simulink model "wb_poco_al_intfract_v00"  (Simulink 6.2)
settings: Solver=ode45  StartTime=0.0  StopTime=2^23  RelTol=1e-3
libraries: xbsIndex_r3 x705, xps_library x24, delay_lib x6, fft_library x2, pfb_library x1
(part 3 of 6)

== system wb_poco_al_intfract_v00/delay_wideband_prog0/delay_dp3 ==
  din : Inport  Port=1  LatchInput=off
  delay : Inport  Port=2  LatchInput=off
  AddSub : xbsIndex_r3/AddSub  mode=Subtraction  precision=User Defined  arith_type=Unsigned  n_bits=11  bin_pt=0  quantization=Truncate  overflow=Wrap  latency=1  explicit_period=off  period=1  use_carryin=off  use_carryout=off  en=off  dbl_ovrd=off  show_param=off  use_core=on  pipeline=off  use_rpm=on  gen_core=off
      settings: xl_area=[0, 0, 0, 0, 0, 0, 0]
  Constant2 : xbsIndex_r3/Constant  const=1  equ=P=C  arith_type=Boolean  n_bits=1  bin_pt=0  opselect=C  inp2=PCIN>>17  opr=+  inp1=P  carry=CIN  iostate=0  explicit_period=on  period=1  dbl_ovrd=off
  Constant4 : xbsIndex_r3/Constant  const=0  equ=P=C  arith_type=Boolean  n_bits=1  bin_pt=0  opselect=C  inp2=PCIN>>17  opr=+  inp1=P  carry=CIN  iostate=0  explicit_period=on  period=1  dbl_ovrd=off
  Dual Port RAM : S-Function  AncestorBlock=xbsIndex_r3/Dual Port RAM  FunctionName=xldpram  Parameters=sfcn_mwsv__  mask(Xilinx Dual Port Random Access Memory){depth=2048, initVector=0, write_mode_A=Read After Write, write_mode_B=Read After Write, latency=4, mem_collision=off, init_zero=on, explicit_period=off, period=1, dbl_ovrd=off, rst_a=off, init_a=0, rst_b=off, init_b=0, show_param=off, distributed_mem=off, use_rpm=off, gen_core=off, xl_area=[0, 0, 0, 0, 0, 0, 0], xl_use_area=off}
      mask prompts: initVector "Initial Value Vector"; write_mode_A "Write Mode:  Port A"; write_mode_B "Write Mode:  Port B"; mem_collision "Provide Output Valid Port"; init_zero "Zero Initial Output  (otherwise NaN)"; explicit_period "Use Explicit Sample Period"; period "Sample Period  (use -1 to inherit first known input period)"; dbl_ovrd "Override with Doubles"; rst_a "Provide Reset Port for Port A Output Register"; init_a "Initial Value for Port A Output Register"; rst_b "Provide Reset Port for Port B Output Register"; init_b "Initial Value for Port B Output Register"; show_param "---------------------- Show Implementation Parameters -----------------------------------------------------------------------------------"; distributed_mem "Use Distributed Memory (instead of block RAM)"; use_rpm "Use Placement Information for Core"; gen_core "Generate Core"; xl_area "FPGA Area [Slices, FFs, BRAMs, LUTs, IOBs, Emb. Mults, TBUFs]"; xl_use_area "Use Area Above For Estimation"
      mask help: Dual port random access memory (RAM). Independent address, data and write enable ports allow shared access to a single memory space. Dual ports enable simultaneous access to the memory space at different sample rates using multiple data widths.
      mask init: same as wb_poco_al_intfract_v00/delay_wideband_prog0/delay_dp/Dual Port RAM
      mask Help: eval('xlWeb(xlhtmldoclink(''Dual Port RAM''))');
      mask StyleString: edit,edit,popup(Read After Write|Read Before Write|No Read On Write),popup(Read After Write|Read Before Write|No Read On Write),edit,checkbox,checkbox,checkbox,edit,checkbox,checkbox,edit,checkbox,edit,checkbox,checkbox,checkbox,checkbox,edit,checkbox
      mask CallbackString: |||||||xldpramCallback|||xldpramCallback||xldpramCallback||xldpramCallback|xldpramCallback||||
      mask Display:
      | patch([0 iWidth iWidth 0],[0 0 iHeight iHeight] ,bg);
      | patch([0 iWidth iWidth 0],[iCy-2 iCy-2 iCy+2 iCy+2] , .9* bg);
      | patch(logoX,logoY , fg);
      | port_label('input',1,'addr_A');
      | port_label('input',2,'data_A');
      | port_label('input',3,'we_A');
      | port_label('input',4,'addr_B');
      | port_label('input',dataBPNum,dataBStr);
      | port_label('input',weBPNum,weBStr);
      | port_label('input',rstAPNum,rstAStr);
      | port_label('input',rstBPNum,rstBStr);
      | port_label('output',1,'A');
      | port_label('output',doutBPNum,'B');
      | port_label('output',voutAPNum,voutAStr);
      | port_label('output',voutBPNum,voutBStr);
      | ;plot([0 0 iWidth iWidth 0], [0 iHeight iHeight 0 0]);
  wr_addr : xbsIndex_r3/Counter  cnt_type=Free Running  n_bits=11  bin_pt=0  arith_type=Unsigned  start_count=0  cnt_to=Inf  cnt_by_val=1  operation=Up  explicit_period=off  period=1  load_pin=off  rst=off  en=off  dbl_ovrd=off  show_param=off  use_rpm=on  gen_core=off
      settings: xl_area=[0, 0, 0, 0, 0, 0, 0]
  dout : Outport
  wires:
  wr_addr/1 -> AddSub/1, Dual Port RAM/1
  Constant2/1 -> Dual Port RAM/3
  din/1 -> Dual Port RAM/5, Dual Port RAM/2
  Constant4/1 -> Dual Port RAM/6
  delay/1 -> AddSub/2
  AddSub/1 -> Dual Port RAM/4
  Dual Port RAM/2 -> dout/1

== system wb_poco_al_intfract_v00/delay_wideband_prog0/sync_delay ==
  In : Inport  Port=1  LatchInput=off
  Constant : xbsIndex_r3/Constant  const=1  equ=P=C  arith_type=Unsigned  n_bits=BitWidth  bin_pt=0  opselect=C  inp2=PCIN>>17  opr=+  inp1=P  carry=CIN  iostate=0  explicit_period=on  period=1  dbl_ovrd=off
  Constant1 : xbsIndex_r3/Constant  const=0  equ=P=C  arith_type=Unsigned  n_bits=BitWidth  bin_pt=0  opselect=C  inp2=PCIN>>17  opr=+  inp1=P  carry=CIN  iostate=0  explicit_period=on  period=1  dbl_ovrd=off
  Constant2 : xbsIndex_r3/Constant  const=DelayLen  equ=P=C  arith_type=Unsigned  n_bits=BitWidth  bin_pt=0  opselect=C  inp2=PCIN>>17  opr=+  inp1=P  carry=CIN  iostate=0  explicit_period=on  period=1  dbl_ovrd=off
  Constant3 : xbsIndex_r3/Constant  const=UseCounter  equ=P=C  arith_type=Unsigned  n_bits=1  bin_pt=0  opselect=C  inp2=PCIN>>17  opr=+  inp1=P  carry=CIN  iostate=0  explicit_period=on  period=1  dbl_ovrd=off
  Counter : xbsIndex_r3/Counter  cnt_type=Free Running  n_bits=BitWidth  bin_pt=0  arith_type=Unsigned  start_count=0  cnt_to=Inf  cnt_by_val=1  operation=Down  explicit_period=on  period=1  load_pin=on  rst=off  en=on  dbl_ovrd=off  show_param=off  use_rpm=on  gen_core=off
      settings: xl_area=[0, 0, 0, 0, 0, 0, 0]
  Logical : xbsIndex_r3/Logical  logical_function=OR  inputs=2  precision=Full  arith_type=Unsigned  n_bits=8  bin_pt=2  align_bp=on  latency=0  explicit_period=on  period=1  en=off  dbl_ovrd=off  show_param=off
      settings: xl_area=[0, 0, 0, 0, 0, 0, 0]
  Mux : xbsIndex_r3/Mux  inputs=2  precision=Full  arith_type="Signed  (2's comp)"  n_bits=8  bin_pt=2  quantization=Truncate  overflow=Wrap  latency=0  explicit_period=off  period=1  en=off  dbl_ovrd=off  show_param=off  mux_type=off  use_rpm=off  gen_core=off
      settings: xl_area=[0, 0, 0, 0, 0, 0, 0]
  Relational : xbsIndex_r3/Relational  mode=a=b  latency=0  explicit_period=off  period=1  en=off  dbl_ovrd=off  show_param=off
      settings: xl_area=[0, 0, 0, 0, 0, 0, 0]
  Relational1 : xbsIndex_r3/Relational  mode=a!=b  latency=0  explicit_period=on  period=1  en=off  dbl_ovrd=off  show_param=off
      settings: xl_area=[0, 0, 0, 0, 0, 0, 0]
  Out : Outport
  wires:
  Counter/1 -> Relational1/1, Relational/2
  Constant1/1 -> Relational1/2
  Constant/1 -> Relational/1
  Constant2/1 -> Counter/2
  In/1 -> Counter/1, Logical/1, Mux/2
  Logical/1 -> Counter/3
  Relational1/1 -> Logical/2
  Relational/1 -> Mux/3
  Constant3/1 -> Mux/1
  Mux/1 -> Out/1

== system wb_poco_al_intfract_v00/delay_wideband_prog1/barrel_switcher ==
  sel : Inport  Port=1  LatchInput=off
  sync_in : Inport  Port=2  LatchInput=off
  In1 : Inport  Port=3  LatchInput=off
  In2 : Inport  Port=4  LatchInput=off
  In3 : Inport  Port=5  LatchInput=off
  In4 : Inport  Port=6  LatchInput=off
  Delay1 : xbsIndex_r3/Delay  latency=1  reg_retiming=off  explicit_period=off  period=1  en=off  accept_only_valid=off  init_zero=on  dbl_ovrd=off  show_param=off
      settings: xl_area=[0, 0, 0, 0, 0, 0, 0]
  Delay_sync : xbsIndex_r3/Delay  latency=2  reg_retiming=off  explicit_period=off  period=1  en=off  accept_only_valid=off  init_zero=on  dbl_ovrd=off  show_param=off
      settings: xl_area=[0, 0, 0, 0, 0, 0, 0]
  Mux{11..12,21..22,31..32,41..42} (8 alike) : xbsIndex_r3/Mux  inputs=2  precision=Full  arith_type="Signed  (2's comp)"  n_bits=8  bin_pt=2  quantization=Truncate  overflow=Wrap  latency=1  explicit_period=off  period=1  en=off  dbl_ovrd=off  show_param=off  mux_type=off  use_rpm=off  gen_core=off
      settings: xl_area=[0, 0, 0, 0, 0, 0, 0]
  Slice1 : xbsIndex_r3/Slice  mode=Upper Bit Location + Width  nbits=1  bit1=-0  base1=MSB of Input  bit0=0  base0=LSB of Input  boolean_output=off  explicit_period=off  period=1  dbl_ovrd=off
  Slice2 : xbsIndex_r3/Slice  mode=Upper Bit Location + Width  nbits=1  bit1=-1  base1=MSB of Input  bit0=0  base0=LSB of Input  boolean_output=off  explicit_period=off  period=1  dbl_ovrd=off
  sync_out : Outport
  Out1 : Outport  Port=2
  Out2 : Outport  Port=3
  Out3 : Outport  Port=4
  Out4 : Outport  Port=5
  wires:
  Mux41/1 -> Mux32/3, Mux42/2
  Mux31/1 -> Mux22/3, Mux32/2
  Mux21/1 -> Mux12/3, Mux22/2
  Mux11/1 -> Mux42/3, Mux12/2
  Mux42/1 -> Out4/1
  In4/1 -> Mux21/3, Mux41/2
  Mux32/1 -> Out3/1
  In3/1 -> Mux11/3, Mux31/2
  Mux22/1 -> Out2/1
  In2/1 -> Mux41/3, Mux21/2
  Mux12/1 -> Out1/1
  In1/1 -> Mux31/3, Mux11/2
  Slice2/1 -> Mux42/1, Mux32/1, Mux22/1, Mux12/1
  Slice1/1 -> Mux41/1, Mux31/1, Mux21/1, Mux11/1
  Delay1/1 -> Slice2/1
  sel/1 -> Delay1/1, Slice1/1
  Delay_sync/1 -> sync_out/1
  sync_in/1 -> Delay_sync/1

== system wb_poco_al_intfract_v00/delay_wideband_prog1/delay_dp ==
  din : Inport  Port=1  LatchInput=off
  delay : Inport  Port=2  LatchInput=off
  AddSub : xbsIndex_r3/AddSub  mode=Subtraction  precision=User Defined  arith_type=Unsigned  n_bits=11  bin_pt=0  quantization=Truncate  overflow=Wrap  latency=1  explicit_period=off  period=1  use_carryin=off  use_carryout=off  en=off  dbl_ovrd=off  show_param=off  use_core=on  pipeline=off  use_rpm=on  gen_core=off
      settings: xl_area=[0, 0, 0, 0, 0, 0, 0]
  Constant2 : xbsIndex_r3/Constant  const=1  equ=P=C  arith_type=Boolean  n_bits=1  bin_pt=0  opselect=C  inp2=PCIN>>17  opr=+  inp1=P  carry=CIN  iostate=0  explicit_period=on  period=1  dbl_ovrd=off
  Constant4 : xbsIndex_r3/Constant  const=0  equ=P=C  arith_type=Boolean  n_bits=1  bin_pt=0  opselect=C  inp2=PCIN>>17  opr=+  inp1=P  carry=CIN  iostate=0  explicit_period=on  period=1  dbl_ovrd=off
  Dual Port RAM : S-Function  AncestorBlock=xbsIndex_r3/Dual Port RAM  FunctionName=xldpram  Parameters=sfcn_mwsv__  mask(Xilinx Dual Port Random Access Memory){depth=2048, initVector=0, write_mode_A=Read After Write, write_mode_B=Read After Write, latency=4, mem_collision=off, init_zero=on, explicit_period=off, period=1, dbl_ovrd=off, rst_a=off, init_a=0, rst_b=off, init_b=0, show_param=off, distributed_mem=off, use_rpm=off, gen_core=off, xl_area=[0, 0, 0, 0, 0, 0, 0], xl_use_area=off}
      mask prompts: initVector "Initial Value Vector"; write_mode_A "Write Mode:  Port A"; write_mode_B "Write Mode:  Port B"; mem_collision "Provide Output Valid Port"; init_zero "Zero Initial Output  (otherwise NaN)"; explicit_period "Use Explicit Sample Period"; period "Sample Period  (use -1 to inherit first known input period)"; dbl_ovrd "Override with Doubles"; rst_a "Provide Reset Port for Port A Output Register"; init_a "Initial Value for Port A Output Register"; rst_b "Provide Reset Port for Port B Output Register"; init_b "Initial Value for Port B Output Register"; show_param "---------------------- Show Implementation Parameters -----------------------------------------------------------------------------------"; distributed_mem "Use Distributed Memory (instead of block RAM)"; use_rpm "Use Placement Information for Core"; gen_core "Generate Core"; xl_area "FPGA Area [Slices, FFs, BRAMs, LUTs, IOBs, Emb. Mults, TBUFs]"; xl_use_area "Use Area Above For Estimation"
      mask help: Dual port random access memory (RAM). Independent address, data and write enable ports allow shared access to a single memory space. Dual ports enable simultaneous access to the memory space at different sample rates using multiple data widths.
      mask init: same as wb_poco_al_intfract_v00/delay_wideband_prog0/delay_dp/Dual Port RAM
      mask Help: eval('xlWeb(xlhtmldoclink(''Dual Port RAM''))');
      mask StyleString: edit,edit,popup(Read After Write|Read Before Write|No Read On Write),popup(Read After Write|Read Before Write|No Read On Write),edit,checkbox,checkbox,checkbox,edit,checkbox,checkbox,edit,checkbox,edit,checkbox,checkbox,checkbox,checkbox,edit,checkbox
      mask CallbackString: |||||||xldpramCallback|||xldpramCallback||xldpramCallback||xldpramCallback|xldpramCallback||||
      mask Display:
      | patch([0 iWidth iWidth 0],[0 0 iHeight iHeight] ,bg);
      | patch([0 iWidth iWidth 0],[iCy-2 iCy-2 iCy+2 iCy+2] , .9* bg);
      | patch(logoX,logoY , fg);
      | port_label('input',1,'addr_A');
      | port_label('input',2,'data_A');
      | port_label('input',3,'we_A');
      | port_label('input',4,'addr_B');
      | port_label('input',dataBPNum,dataBStr);
      | port_label('input',weBPNum,weBStr);
      | port_label('input',rstAPNum,rstAStr);
      | port_label('input',rstBPNum,rstBStr);
      | port_label('output',1,'A');
      | port_label('output',doutBPNum,'B');
      | port_label('output',voutAPNum,voutAStr);
      | port_label('output',voutBPNum,voutBStr);
      | ;plot([0 0 iWidth iWidth 0], [0 iHeight iHeight 0 0]);
  wr_addr : xbsIndex_r3/Counter  cnt_type=Free Running  n_bits=11  bin_pt=0  arith_type=Unsigned  start_count=0  cnt_to=Inf  cnt_by_val=1  operation=Up  explicit_period=off  period=1  load_pin=off  rst=off  en=off  dbl_ovrd=off  show_param=off  use_rpm=on  gen_core=off
      settings: xl_area=[0, 0, 0, 0, 0, 0, 0]
  dout : Outport
  wires:
  wr_addr/1 -> AddSub/1, Dual Port RAM/1
  Constant2/1 -> Dual Port RAM/3
  din/1 -> Dual Port RAM/5, Dual Port RAM/2
  Constant4/1 -> Dual Port RAM/6
  delay/1 -> AddSub/2
  AddSub/1 -> Dual Port RAM/4
  Dual Port RAM/2 -> dout/1

== system wb_poco_al_intfract_v00/delay_wideband_prog1/delay_dp1 ==
  din : Inport  Port=1  LatchInput=off
  delay : Inport  Port=2  LatchInput=off
  AddSub : xbsIndex_r3/AddSub  mode=Subtraction  precision=User Defined  arith_type=Unsigned  n_bits=11  bin_pt=0  quantization=Truncate  overflow=Wrap  latency=1  explicit_period=off  period=1  use_carryin=off  use_carryout=off  en=off  dbl_ovrd=off  show_param=off  use_core=on  pipeline=off  use_rpm=on  gen_core=off
      settings: xl_area=[0, 0, 0, 0, 0, 0, 0]
  Constant2 : xbsIndex_r3/Constant  const=1  equ=P=C  arith_type=Boolean  n_bits=1  bin_pt=0  opselect=C  inp2=PCIN>>17  opr=+  inp1=P  carry=CIN  iostate=0  explicit_period=on  period=1  dbl_ovrd=off
  Constant4 : xbsIndex_r3/Constant  const=0  equ=P=C  arith_type=Boolean  n_bits=1  bin_pt=0  opselect=C  inp2=PCIN>>17  opr=+  inp1=P  carry=CIN  iostate=0  explicit_period=on  period=1  dbl_ovrd=off
  Dual Port RAM : S-Function  AncestorBlock=xbsIndex_r3/Dual Port RAM  FunctionName=xldpram  Parameters=sfcn_mwsv__  mask(Xilinx Dual Port Random Access Memory){depth=2048, initVector=0, write_mode_A=Read After Write, write_mode_B=Read After Write, latency=4, mem_collision=off, init_zero=on, explicit_period=off, period=1, dbl_ovrd=off, rst_a=off, init_a=0, rst_b=off, init_b=0, show_param=off, distributed_mem=off, use_rpm=off, gen_core=off, xl_area=[0, 0, 0, 0, 0, 0, 0], xl_use_area=off}
      mask prompts: initVector "Initial Value Vector"; write_mode_A "Write Mode:  Port A"; write_mode_B "Write Mode:  Port B"; mem_collision "Provide Output Valid Port"; init_zero "Zero Initial Output  (otherwise NaN)"; explicit_period "Use Explicit Sample Period"; period "Sample Period  (use -1 to inherit first known input period)"; dbl_ovrd "Override with Doubles"; rst_a "Provide Reset Port for Port A Output Register"; init_a "Initial Value for Port A Output Register"; rst_b "Provide Reset Port for Port B Output Register"; init_b "Initial Value for Port B Output Register"; show_param "---------------------- Show Implementation Parameters -----------------------------------------------------------------------------------"; distributed_mem "Use Distributed Memory (instead of block RAM)"; use_rpm "Use Placement Information for Core"; gen_core "Generate Core"; xl_area "FPGA Area [Slices, FFs, BRAMs, LUTs, IOBs, Emb. Mults, TBUFs]"; xl_use_area "Use Area Above For Estimation"
      mask help: Dual port random access memory (RAM). Independent address, data and write enable ports allow shared access to a single memory space. Dual ports enable simultaneous access to the memory space at different sample rates using multiple data widths.
      mask init: same as wb_poco_al_intfract_v00/delay_wideband_prog0/delay_dp/Dual Port RAM
      mask Help: eval('xlWeb(xlhtmldoclink(''Dual Port RAM''))');
      mask StyleString: edit,edit,popup(Read After Write|Read Before Write|No Read On Write),popup(Read After Write|Read Before Write|No Read On Write),edit,checkbox,checkbox,checkbox,edit,checkbox,checkbox,edit,checkbox,edit,checkbox,checkbox,checkbox,checkbox,edit,checkbox
      mask CallbackString: |||||||xldpramCallback|||xldpramCallback||xldpramCallback||xldpramCallback|xldpramCallback||||
      mask Display:
      | patch([0 iWidth iWidth 0],[0 0 iHeight iHeight] ,bg);
      | patch([0 iWidth iWidth 0],[iCy-2 iCy-2 iCy+2 iCy+2] , .9* bg);
      | patch(logoX,logoY , fg);
      | port_label('input',1,'addr_A');
      | port_label('input',2,'data_A');
      | port_label('input',3,'we_A');
      | port_label('input',4,'addr_B');
      | port_label('input',dataBPNum,dataBStr);
      | port_label('input',weBPNum,weBStr);
      | port_label('input',rstAPNum,rstAStr);
      | port_label('input',rstBPNum,rstBStr);
      | port_label('output',1,'A');
      | port_label('output',doutBPNum,'B');
      | port_label('output',voutAPNum,voutAStr);
      | port_label('output',voutBPNum,voutBStr);
      | ;plot([0 0 iWidth iWidth 0], [0 iHeight iHeight 0 0]);
  wr_addr : xbsIndex_r3/Counter  cnt_type=Free Running  n_bits=11  bin_pt=0  arith_type=Unsigned  start_count=0  cnt_to=Inf  cnt_by_val=1  operation=Up  explicit_period=off  period=1  load_pin=off  rst=off  en=off  dbl_ovrd=off  show_param=off  use_rpm=on  gen_core=off
      settings: xl_area=[0, 0, 0, 0, 0, 0, 0]
  dout : Outport
  wires:
  Dual Port RAM/2 -> dout/1
  AddSub/1 -> Dual Port RAM/4
  delay/1 -> AddSub/2
  Constant4/1 -> Dual Port RAM/6
  din/1 -> Dual Port RAM/2, Dual Port RAM/5
  Constant2/1 -> Dual Port RAM/3
  wr_addr/1 -> Dual Port RAM/1, AddSub/1

== system wb_poco_al_intfract_v00/delay_wideband_prog1/delay_dp2 ==
  din : Inport  Port=1  LatchInput=off
  delay : Inport  Port=2  LatchInput=off
  AddSub : xbsIndex_r3/AddSub  mode=Subtraction  precision=User Defined  arith_type=Unsigned  n_bits=11  bin_pt=0  quantization=Truncate  overflow=Wrap  latency=1  explicit_period=off  period=1  use_carryin=off  use_carryout=off  en=off  dbl_ovrd=off  show_param=off  use_core=on  pipeline=off  use_rpm=on  gen_core=off
      settings: xl_area=[0, 0, 0, 0, 0, 0, 0]
  Constant2 : xbsIndex_r3/Constant  const=1  equ=P=C  arith_type=Boolean  n_bits=1  bin_pt=0  opselect=C  inp2=PCIN>>17  opr=+  inp1=P  carry=CIN  iostate=0  explicit_period=on  period=1  dbl_ovrd=off
  Constant4 : xbsIndex_r3/Constant  const=0  equ=P=C  arith_type=Boolean  n_bits=1  bin_pt=0  opselect=C  inp2=PCIN>>17  opr=+  inp1=P  carry=CIN  iostate=0  explicit_period=on  period=1  dbl_ovrd=off
  Dual Port RAM : S-Function  AncestorBlock=xbsIndex_r3/Dual Port RAM  FunctionName=xldpram  Parameters=sfcn_mwsv__  mask(Xilinx Dual Port Random Access Memory){depth=2048, initVector=0, write_mode_A=Read After Write, write_mode_B=Read After Write, latency=4, mem_collision=off, init_zero=on, explicit_period=off, period=1, dbl_ovrd=off, rst_a=off, init_a=0, rst_b=off, init_b=0, show_param=off, distributed_mem=off, use_rpm=off, gen_core=off, xl_area=[0, 0, 0, 0, 0, 0, 0], xl_use_area=off}
      mask prompts: initVector "Initial Value Vector"; write_mode_A "Write Mode:  Port A"; write_mode_B "Write Mode:  Port B"; mem_collision "Provide Output Valid Port"; init_zero "Zero Initial Output  (otherwise NaN)"; explicit_period "Use Explicit Sample Period"; period "Sample Period  (use -1 to inherit first known input period)"; dbl_ovrd "Override with Doubles"; rst_a "Provide Reset Port for Port A Output Register"; init_a "Initial Value for Port A Output Register"; rst_b "Provide Reset Port for Port B Output Register"; init_b "Initial Value for Port B Output Register"; show_param "---------------------- Show Implementation Parameters -----------------------------------------------------------------------------------"; distributed_mem "Use Distributed Memory (instead of block RAM)"; use_rpm "Use Placement Information for Core"; gen_core "Generate Core"; xl_area "FPGA Area [Slices, FFs, BRAMs, LUTs, IOBs, Emb. Mults, TBUFs]"; xl_use_area "Use Area Above For Estimation"
      mask help: Dual port random access memory (RAM). Independent address, data and write enable ports allow shared access to a single memory space. Dual ports enable simultaneous access to the memory space at different sample rates using multiple data widths.
      mask init: same as wb_poco_al_intfract_v00/delay_wideband_prog0/delay_dp/Dual Port RAM
      mask Help: eval('xlWeb(xlhtmldoclink(''Dual Port RAM''))');
      mask StyleString: edit,edit,popup(Read After Write|Read Before Write|No Read On Write),popup(Read After Write|Read Before Write|No Read On Write),edit,checkbox,checkbox,checkbox,edit,checkbox,checkbox,edit,checkbox,edit,checkbox,checkbox,checkbox,checkbox,edit,checkbox
      mask CallbackString: |||||||xldpramCallback|||xldpramCallback||xldpramCallback||xldpramCallback|xldpramCallback||||
      mask Display:
      | patch([0 iWidth iWidth 0],[0 0 iHeight iHeight] ,bg);
      | patch([0 iWidth iWidth 0],[iCy-2 iCy-2 iCy+2 iCy+2] , .9* bg);
      | patch(logoX,logoY , fg);
      | port_label('input',1,'addr_A');
      | port_label('input',2,'data_A');
      | port_label('input',3,'we_A');
      | port_label('input',4,'addr_B');
      | port_label('input',dataBPNum,dataBStr);
      | port_label('input',weBPNum,weBStr);
      | port_label('input',rstAPNum,rstAStr);
      | port_label('input',rstBPNum,rstBStr);
      | port_label('output',1,'A');
      | port_label('output',doutBPNum,'B');
      | port_label('output',voutAPNum,voutAStr);
      | port_label('output',voutBPNum,voutBStr);
      | ;plot([0 0 iWidth iWidth 0], [0 iHeight iHeight 0 0]);
  wr_addr : xbsIndex_r3/Counter  cnt_type=Free Running  n_bits=11  bin_pt=0  arith_type=Unsigned  start_count=0  cnt_to=Inf  cnt_by_val=1  operation=Up  explicit_period=off  period=1  load_pin=off  rst=off  en=off  dbl_ovrd=off  show_param=off  use_rpm=on  gen_core=off
      settings: xl_area=[0, 0, 0, 0, 0, 0, 0]
  dout : Outport
  wires:
  wr_addr/1 -> AddSub/1, Dual Port RAM/1
  Constant2/1 -> Dual Port RAM/3
  din/1 -> Dual Port RAM/5, Dual Port RAM/2
  Constant4/1 -> Dual Port RAM/6
  delay/1 -> AddSub/2
  AddSub/1 -> Dual Port RAM/4
  Dual Port RAM/2 -> dout/1

== system wb_poco_al_intfract_v00/delay_wideband_prog1/delay_dp3 ==
  din : Inport  Port=1  LatchInput=off
  delay : Inport  Port=2  LatchInput=off
  AddSub : xbsIndex_r3/AddSub  mode=Subtraction  precision=User Defined  arith_type=Unsigned  n_bits=11  bin_pt=0  quantization=Truncate  overflow=Wrap  latency=1  explicit_period=off  period=1  use_carryin=off  use_carryout=off  en=off  dbl_ovrd=off  show_param=off  use_core=on  pipeline=off  use_rpm=on  gen_core=off
      settings: xl_area=[0, 0, 0, 0, 0, 0, 0]
  Constant2 : xbsIndex_r3/Constant  const=1  equ=P=C  arith_type=Boolean  n_bits=1  bin_pt=0  opselect=C  inp2=PCIN>>17  opr=+  inp1=P  carry=CIN  iostate=0  explicit_period=on  period=1  dbl_ovrd=off
  Constant4 : xbsIndex_r3/Constant  const=0  equ=P=C  arith_type=Boolean  n_bits=1  bin_pt=0  opselect=C  inp2=PCIN>>17  opr=+  inp1=P  carry=CIN  iostate=0  explicit_period=on  period=1  dbl_ovrd=off
  Dual Port RAM : S-Function  AncestorBlock=xbsIndex_r3/Dual Port RAM  FunctionName=xldpram  Parameters=sfcn_mwsv__  mask(Xilinx Dual Port Random Access Memory){depth=2048, initVector=0, write_mode_A=Read After Write, write_mode_B=Read After Write, latency=4, mem_collision=off, init_zero=on, explicit_period=off, period=1, dbl_ovrd=off, rst_a=off, init_a=0, rst_b=off, init_b=0, show_param=off, distributed_mem=off, use_rpm=off, gen_core=off, xl_area=[0, 0, 0, 0, 0, 0, 0], xl_use_area=off}
      mask prompts: initVector "Initial Value Vector"; write_mode_A "Write Mode:  Port A"; write_mode_B "Write Mode:  Port B"; mem_collision "Provide Output Valid Port"; init_zero "Zero Initial Output  (otherwise NaN)"; explicit_period "Use Explicit Sample Period"; period "Sample Period  (use -1 to inherit first known input period)"; dbl_ovrd "Override with Doubles"; rst_a "Provide Reset Port for Port A Output Register"; init_a "Initial Value for Port A Output Register"; rst_b "Provide Reset Port for Port B Output Register"; init_b "Initial Value for Port B Output Register"; show_param "---------------------- Show Implementation Parameters -----------------------------------------------------------------------------------"; distributed_mem "Use Distributed Memory (instead of block RAM)"; use_rpm "Use Placement Information for Core"; gen_core "Generate Core"; xl_area "FPGA Area [Slices, FFs, BRAMs, LUTs, IOBs, Emb. Mults, TBUFs]"; xl_use_area "Use Area Above For Estimation"
      mask help: Dual port random access memory (RAM). Independent address, data and write enable ports allow shared access to a single memory space. Dual ports enable simultaneous access to the memory space at different sample rates using multiple data widths.
      mask init: same as wb_poco_al_intfract_v00/delay_wideband_prog0/delay_dp/Dual Port RAM
      mask Help: eval('xlWeb(xlhtmldoclink(''Dual Port RAM''))');
      mask StyleString: edit,edit,popup(Read After Write|Read Before Write|No Read On Write),popup(Read After Write|Read Before Write|No Read On Write),edit,checkbox,checkbox,checkbox,edit,checkbox,checkbox,edit,checkbox,edit,checkbox,checkbox,checkbox,checkbox,edit,checkbox
      mask CallbackString: |||||||xldpramCallback|||xldpramCallback||xldpramCallback||xldpramCallback|xldpramCallback||||
      mask Display:
      | patch([0 iWidth iWidth 0],[0 0 iHeight iHeight] ,bg);
      | patch([0 iWidth iWidth 0],[iCy-2 iCy-2 iCy+2 iCy+2] , .9* bg);
      | patch(logoX,logoY , fg);
      | port_label('input',1,'addr_A');
      | port_label('input',2,'data_A');
      | port_label('input',3,'we_A');
      | port_label('input',4,'addr_B');
      | port_label('input',dataBPNum,dataBStr);
      | port_label('input',weBPNum,weBStr);
      | port_label('input',rstAPNum,rstAStr);
      | port_label('input',rstBPNum,rstBStr);
      | port_label('output',1,'A');
      | port_label('output',doutBPNum,'B');
      | port_label('output',voutAPNum,voutAStr);
      | port_label('output',voutBPNum,voutBStr);
      | ;plot([0 0 iWidth iWidth 0], [0 iHeight iHeight 0 0]);
  wr_addr : xbsIndex_r3/Counter  cnt_type=Free Running  n_bits=11  bin_pt=0  arith_type=Unsigned  start_count=0  cnt_to=Inf  cnt_by_val=1  operation=Up  explicit_period=off  period=1  load_pin=off  rst=off  en=off  dbl_ovrd=off  show_param=off  use_rpm=on  gen_core=off
      settings: xl_area=[0, 0, 0, 0, 0, 0, 0]
  dout : Outport
  wires:
  Dual Port RAM/2 -> dout/1
  AddSub/1 -> Dual Port RAM/4
  delay/1 -> AddSub/2
  Constant4/1 -> Dual Port RAM/6
  din/1 -> Dual Port RAM/2, Dual Port RAM/5
  Constant2/1 -> Dual Port RAM/3
  wr_addr/1 -> Dual Port RAM/1, AddSub/1

== system wb_poco_al_intfract_v00/delay_wideband_prog1/sync_delay ==
  In : Inport  Port=1  LatchInput=off
  Constant : xbsIndex_r3/Constant  const=1  equ=P=C  arith_type=Unsigned  n_bits=BitWidth  bin_pt=0  opselect=C  inp2=PCIN>>17  opr=+  inp1=P  carry=CIN  iostate=0  explicit_period=on  period=1  dbl_ovrd=off
  Constant1 : xbsIndex_r3/Constant  const=0  equ=P=C  arith_type=Unsigned  n_bits=BitWidth  bin_pt=0  opselect=C  inp2=PCIN>>17  opr=+  inp1=P  carry=CIN  iostate=0  explicit_period=on  period=1  dbl_ovrd=off
  Constant2 : xbsIndex_r3/Constant  const=DelayLen  equ=P=C  arith_type=Unsigned  n_bits=BitWidth  bin_pt=0  opselect=C  inp2=PCIN>>17  opr=+  inp1=P  carry=CIN  iostate=0  explicit_period=on  period=1  dbl_ovrd=off
  Constant3 : xbsIndex_r3/Constant  const=UseCounter  equ=P=C  arith_type=Unsigned  n_bits=1  bin_pt=0  opselect=C  inp2=PCIN>>17  opr=+  inp1=P  carry=CIN  iostate=0  explicit_period=on  period=1  dbl_ovrd=off
  Counter : xbsIndex_r3/Counter  cnt_type=Free Running  n_bits=BitWidth  bin_pt=0  arith_type=Unsigned  start_count=0  cnt_to=Inf  cnt_by_val=1  operation=Down  explicit_period=on  period=1  load_pin=on  rst=off  en=on  dbl_ovrd=off  show_param=off  use_rpm=on  gen_core=off
      settings: xl_area=[0, 0, 0, 0, 0, 0, 0]
  Logical : xbsIndex_r3/Logical  logical_function=OR  inputs=2  precision=Full  arith_type=Unsigned  n_bits=8  bin_pt=2  align_bp=on  latency=0  explicit_period=on  period=1  en=off  dbl_ovrd=off  show_param=off
      settings: xl_area=[0, 0, 0, 0, 0, 0, 0]
  Mux : xbsIndex_r3/Mux  inputs=2  precision=Full  arith_type="Signed  (2's comp)"  n_bits=8  bin_pt=2  quantization=Truncate  overflow=Wrap  latency=0  explicit_period=off  period=1  en=off  dbl_ovrd=off  show_param=off  mux_type=off  use_rpm=off  gen_core=off
      settings: xl_area=[0, 0, 0, 0, 0, 0, 0]
  Relational : xbsIndex_r3/Relational  mode=a=b  latency=0  explicit_period=off  period=1  en=off  dbl_ovrd=off  show_param=off
      settings: xl_area=[0, 0, 0, 0, 0, 0, 0]
  Relational1 : xbsIndex_r3/Relational  mode=a!=b  latency=0  explicit_period=on  period=1  en=off  dbl_ovrd=off  show_param=off
      settings: xl_area=[0, 0, 0, 0, 0, 0, 0]
  Out : Outport
  wires:
  Mux/1 -> Out/1
  Constant3/1 -> Mux/1
  Relational/1 -> Mux/3
  Relational1/1 -> Logical/2
  Logical/1 -> Counter/3
  In/1 -> Mux/2, Logical/1, Counter/1
  Constant2/1 -> Counter/2
  Constant/1 -> Relational/1
  Constant1/1 -> Relational1/2
  Counter/1 -> Relational/2, Relational1/1

== system wb_poco_al_intfract_v00/dir_x/aa ==
  a+bi : Inport  Port=1  LatchInput=off
  c+di : Inport  Port=2  LatchInput=off
  new_acc : Inport  Port=3  LatchInput=off
  Counter : xbsIndex_r3/Counter  cnt_type=Free Running  n_bits=chan_bits  bin_pt=0  arith_type=Unsigned  start_count=0  cnt_to=Inf  cnt_by_val=1  operation=Up  explicit_period=off  period=1  load_pin=off  rst=on  en=on  dbl_ovrd=off  show_param=off  use_rpm=on  gen_core=off
      settings: xl_area=[0, 0, 0, 0, 0, 0, 0]
  Delay3 : xbsIndex_r3/Delay  latency=5  reg_retiming=off  explicit_period=off  period=1  en=off  accept_only_valid=off  init_zero=on  dbl_ovrd=off  show_param=off
      settings: xl_area=[0, 0, 0, 0, 0, 0, 0]
  Gateway Out{,1..3} (4 alike) : xbsIndex_r3/Gateway Out  output_type=Double  nbits=8  bin_pt=6  arith_type=Boolean  quantization=Truncate  overflow=Wrap  hdl_port=on  timing_constraint=None  locs_specified=off  LOCs={}  needs_fixed_name=off  show_param=off
      settings: xl_area=[0, 0, 0, 0, 0, 0, 0]
  Reinterpret : xbsIndex_r3/Reinterpret  force_arith_type=on  arith_type=Unsigned  force_bin_pt=on  bin_pt=0  force_valid=on
  Scope : Scope  NumInputPorts=4
      settings: YMin=-1~-1~-1~-1  YMax=1~1~1~1
  Terminator : Terminator
  c_to_ri : Subsystem  mask(Complex to Real-Imag){n_bits=4, bin_pt=3}
      mask prompts: n_bits "Bit Width"; bin_pt "Binary Point"
      mask help: Outputs real and imaginary components of a complex input.
      mask init:
      | annotation=sprintf('%d_%d r/i',n_bits,bin_pt);
      | set_param(gcb,'AttributesFormatString',annotation);
      settings: AttributesFormatString=4_3 r/i
      mask Help:
      | <pre>
      | Description::
      | 
      | Outputs real and imaginary components of a complex input.
      | Useful for simplifying interconnects.
      | See also: Real-Imag to Complex (ri_to_c)
      | 
      | Mask Parameters::
      | 
      | Bit Width (n_bits): Specifies the width of the real/imaginary components.
      | Assumed equal for both components.
      | 
      | Binary Point (bin_pt): Specifies the binary point location in the real/imaginary components.
      | Assumed equal for both components.
      | </pre>
  c_to_ri1 : Subsystem  mask(Complex to Real-Imag){n_bits=4, bin_pt=3}
      mask prompts: n_bits "Bit Width"; bin_pt "Binary Point"
      mask help: Outputs real and imaginary components of a complex input.
      mask init:
      | annotation=sprintf('%d_%d r/i',n_bits,bin_pt);
      | set_param(gcb,'AttributesFormatString',annotation);
      settings: AttributesFormatString=4_3 r/i
      mask Help:
      | <pre>
      | Description::
      | 
      | Outputs real and imaginary components of a complex input.
      | Useful for simplifying interconnects.
      | See also: Real-Imag to Complex (ri_to_c)
      | 
      | Mask Parameters::
      | 
      | Bit Width (n_bits): Specifies the width of the real/imaginary components.
      | Assumed equal for both components.
      | 
      | Binary Point (bin_pt): Specifies the binary point location in the real/imaginary components.
      | Assumed equal for both components.
      | </pre>
  cmult_4bit_br* : Subsystem  mask(cmult_4bit_br*){mult_latency=3, add_latency=2}
      mask prompts: mult_latency "Mult Latency"; add_latency "Add Latency"
      mask help: Perform a conjugating complex multiplication (a+bi)(c-di)=(ac+bd)+(bc-ad)i. Implements the logic in Block RAM.
      mask Help: eval('xlWeb([getenv(''MLIB_ROOT''), ''\doc\html\sp_cmult_4bit_br_\sp_cmult_4bit_br_.html''])')
  real : xps_library/Shared BRAM  Tag=xps:bram  arith_type=Unsigned  addr_width=chan_bits+1  data_width=32  data_bin_pt=0  init_vals=0  sample_rate=1
  vacc_32bit : Subsystem  mask{n_chans=n_chans}
      mask prompts: n_chans "Number of channels"
      mask init:
      | chan_bits=ceil(log2(n_chans));
  wires:
  Reinterpret/1 -> real/2, Gateway Out1/1
  Counter/1 -> real/1, Gateway Out/1
  vacc_32bit/2(valid) -> Counter/2, real/3, Gateway Out2/1
  Delay3/1 -> Counter/1, vacc_32bit/2(new_acc), Gateway Out3/1
  c+di/1 -> c_to_ri1/1(c)
  a+bi/1 -> c_to_ri/1(c)
  c_to_ri1/2(im) -> cmult_4bit_br*/4(d)
  c_to_ri1/1(re) -> cmult_4bit_br*/3(c)
  c_to_ri/2(im) -> cmult_4bit_br*/2(b)
  c_to_ri/1(re) -> cmult_4bit_br*/1(a)
  vacc_32bit/1(dout) -> Reinterpret/1
  new_acc/1 -> Delay3/1
  cmult_4bit_br*/1(real) -> vacc_32bit/1(din)
  real/1 -> Terminator/1
  Gateway Out/1 -> Scope/1
  Gateway Out1/1 -> Scope/2
  Gateway Out2/1 -> Scope/3
  Gateway Out3/1 -> Scope/4

== system wb_poco_al_intfract_v00/dir_x/ac ==
  a+bi : Inport  Port=1  LatchInput=off
  c+di : Inport  Port=2  LatchInput=off
  new_acc : Inport  Port=3  LatchInput=off
  Counter : xbsIndex_r3/Counter  cnt_type=Free Running  n_bits=11  bin_pt=0  arith_type=Unsigned  start_count=0  cnt_to=Inf  cnt_by_val=1  operation=Up  explicit_period=off  period=1  load_pin=off  rst=on  en=on  dbl_ovrd=off  show_param=off  use_rpm=on  gen_core=off
      settings: xl_area=[0, 0, 0, 0, 0, 0, 0]
  Delay3 : xbsIndex_r3/Delay  latency=5  reg_retiming=off  explicit_period=off  period=1  en=off  accept_only_valid=off  init_zero=on  dbl_ovrd=off  show_param=off
      settings: xl_area=[0, 0, 0, 0, 0, 0, 0]
  Reinterpret : xbsIndex_r3/Reinterpret  force_arith_type=on  arith_type=Unsigned  force_bin_pt=on  bin_pt=0  force_valid=on
  Reinterpret1 : xbsIndex_r3/Reinterpret  force_arith_type=on  arith_type=Unsigned  force_bin_pt=on  bin_pt=0  force_valid=on
  c_to_ri : Subsystem  mask(Complex to Real-Imag){n_bits=4, bin_pt=3}
      mask prompts: n_bits "Bit Width"; bin_pt "Binary Point"
      mask help: Outputs real and imaginary components of a complex input.
      mask init:
      | annotation=sprintf('%d_%d r/i',n_bits,bin_pt);
      | set_param(gcb,'AttributesFormatString',annotation);
      settings: AttributesFormatString=4_3 r/i
      mask Help:
      | <pre>
      | Description::
      | 
      | Outputs real and imaginary components of a complex input.
      | Useful for simplifying interconnects.
      | See also: Real-Imag to Complex (ri_to_c)
      | 
      | Mask Parameters::
      | 
      | Bit Width (n_bits): Specifies the width of the real/imaginary components.
      | Assumed equal for both components.
      | 
      | Binary Point (bin_pt): Specifies the binary point location in the real/imaginary components.
      | Assumed equal for both components.
      | </pre>
  c_to_ri1 : Subsystem  mask(Complex to Real-Imag){n_bits=4, bin_pt=3}
      mask prompts: n_bits "Bit Width"; bin_pt "Binary Point"
      mask help: Outputs real and imaginary components of a complex input.
      mask init:
      | annotation=sprintf('%d_%d r/i',n_bits,bin_pt);
      | set_param(gcb,'AttributesFormatString',annotation);
      settings: AttributesFormatString=4_3 r/i
      mask Help:
      | <pre>
      | Description::
      | 
      | Outputs real and imaginary components of a complex input.
      | Useful for simplifying interconnects.
      | See also: Real-Imag to Complex (ri_to_c)
      | 
      | Mask Parameters::
      | 
      | Bit Width (n_bits): Specifies the width of the real/imaginary components.
      | Assumed equal for both components.
      | 
      | Binary Point (bin_pt): Specifies the binary point location in the real/imaginary components.
      | Assumed equal for both components.
      | </pre>
  cmult_4bit_sl* : Subsystem  mask(cmult_4bit_sl*){mult_latency=3, add_latency=2}
      mask prompts: mult_latency "Mult Latency"; add_latency "Add Latency"
      mask help: Perform a conjugating complex multiplication (a+bi)(c-di)=(ac+bd)+(bc-ad)i. Implements the logic in Slices.
      mask Help: eval('xlWeb([getenv(''MLIB_ROOT''), ''\doc\html\sp_cmult_4bit_sl_\sp_cmult_4bit_sl_.html''])')
  imag : xps_library/Shared BRAM  Tag=xps:bram  arith_type=Unsigned  addr_width=chan_bits+1  data_width=32  data_bin_pt=0  init_vals=0  sample_rate=1
  real : xps_library/Shared BRAM  Tag=xps:bram  arith_type=Unsigned  addr_width=chan_bits+1  data_width=32  data_bin_pt=0  init_vals=0  sample_rate=1
  vacc_0 : Subsystem  mask{n_chans=n_chans}
      mask prompts: n_chans "Number of channels"
      mask init:
      | chan_bits=ceil(log2(n_chans));
  vacc_1 : Subsystem  mask{n_chans=n_chans}
      mask prompts: n_chans "Number of channels"
      mask init:
      | chan_bits=ceil(log2(n_chans));
  wires:
  cmult_4bit_sl*/1(real) -> vacc_0/1(din)
  cmult_4bit_sl*/2(imag) -> vacc_1/1(din)
  c_to_ri/1(re) -> cmult_4bit_sl*/1(a)
  c_to_ri/2(im) -> cmult_4bit_sl*/2(b)
  c_to_ri1/1(re) -> cmult_4bit_sl*/3(c)
  c_to_ri1/2(im) -> cmult_4bit_sl*/4(d)
  a+bi/1 -> c_to_ri/1(c)
  c+di/1 -> c_to_ri1/1(c)
  Delay3/1 -> Counter/1, vacc_0/2(new_acc), vacc_1/2(new_acc)
  new_acc/1 -> Delay3/1
  vacc_0/1(dout) -> Reinterpret/1
  vacc_0/2(valid) -> Counter/2, real/3
  Reinterpret/1 -> real/2
  vacc_1/2(valid) -> imag/3
  Reinterpret1/1 -> imag/2
  vacc_1/1(dout) -> Reinterpret1/1
  Counter/1 -> imag/1, real/1

== system wb_poco_al_intfract_v00/dir_x/bb ==
  a+bi : Inport  Port=1  LatchInput=off
  c+di : Inport  Port=2  LatchInput=off
  new_acc : Inport  Port=3  LatchInput=off
  Counter : xbsIndex_r3/Counter  cnt_type=Free Running  n_bits=11  bin_pt=0  arith_type=Unsigned  start_count=0  cnt_to=Inf  cnt_by_val=1  operation=Up  explicit_period=off  period=1  load_pin=off  rst=on  en=on  dbl_ovrd=off  show_param=off  use_rpm=on  gen_core=off
      settings: xl_area=[0, 0, 0, 0, 0, 0, 0]
  Delay3 : xbsIndex_r3/Delay  latency=5  reg_retiming=off  explicit_period=off  period=1  en=off  accept_only_valid=off  init_zero=on  dbl_ovrd=off  show_param=off
      settings: xl_area=[0, 0, 0, 0, 0, 0, 0]
  Reinterpret : xbsIndex_r3/Reinterpret  force_arith_type=on  arith_type=Unsigned  force_bin_pt=on  bin_pt=0  force_valid=on
  c_to_ri : Subsystem  mask(Complex to Real-Imag){n_bits=4, bin_pt=3}
      mask prompts: n_bits "Bit Width"; bin_pt "Binary Point"
      mask help: Outputs real and imaginary components of a complex input.
      mask init:
      | annotation=sprintf('%d_%d r/i',n_bits,bin_pt);
      | set_param(gcb,'AttributesFormatString',annotation);
      settings: AttributesFormatString=4_3 r/i
      mask Help:
      | <pre>
      | Description::
      | 
      | Outputs real and imaginary components of a complex input.
      | Useful for simplifying interconnects.
      | See also: Real-Imag to Complex (ri_to_c)
      | 
      | Mask Parameters::
      | 
      | Bit Width (n_bits): Specifies the width of the real/imaginary components.
      | Assumed equal for both components.
      | 
      | Binary Point (bin_pt): Specifies the binary point location in the real/imaginary components.
      | Assumed equal for both components.
      | </pre>
  c_to_ri1 : Subsystem  mask(Complex to Real-Imag){n_bits=4, bin_pt=3}
      mask prompts: n_bits "Bit Width"; bin_pt "Binary Point"
      mask help: Outputs real and imaginary components of a complex input.
      mask init:
      | annotation=sprintf('%d_%d r/i',n_bits,bin_pt);
      | set_param(gcb,'AttributesFormatString',annotation);
      settings: AttributesFormatString=4_3 r/i
      mask Help:
      | <pre>
      | Description::
      | 
      | Outputs real and imaginary components of a complex input.
      | Useful for simplifying interconnects.
      | See also: Real-Imag to Complex (ri_to_c)
      | 
      | Mask Parameters::
      | 
      | Bit Width (n_bits): Specifies the width of the real/imaginary components.
      | Assumed equal for both components.
      | 
      | Binary Point (bin_pt): Specifies the binary point location in the real/imaginary components.
      | Assumed equal for both components.
      | </pre>
  cmult_4bit_br* : Subsystem  mask(cmult_4bit_br*){mult_latency=3, add_latency=2}
      mask prompts: mult_latency "Mult Latency"; add_latency "Add Latency"
      mask help: Perform a conjugating complex multiplication (a+bi)(c-di)=(ac+bd)+(bc-ad)i. Implements the logic in Block RAM.
      mask Help: eval('xlWeb([getenv(''MLIB_ROOT''), ''\doc\html\sp_cmult_4bit_br_\sp_cmult_4bit_br_.html''])')
  real : xps_library/Shared BRAM  Tag=xps:bram  arith_type=Unsigned  addr_width=chan_bits+1  data_width=32  data_bin_pt=0  init_vals=0  sample_rate=1
  vacc_32bit : Subsystem  mask{n_chans=n_chans}
      mask prompts: n_chans "Number of channels"
      mask init:
      | chan_bits=ceil(log2(n_chans));
  wires:
  cmult_4bit_br*/1(real) -> vacc_32bit/1(din)
  new_acc/1 -> Delay3/1
  vacc_32bit/1(dout) -> Reinterpret/1
  c_to_ri/1(re) -> cmult_4bit_br*/1(a)
  c_to_ri/2(im) -> cmult_4bit_br*/2(b)
  c_to_ri1/1(re) -> cmult_4bit_br*/3(c)
  c_to_ri1/2(im) -> cmult_4bit_br*/4(d)
  a+bi/1 -> c_to_ri/1(c)
  c+di/1 -> c_to_ri1/1(c)
  Delay3/1 -> Counter/1, vacc_32bit/2(new_acc)
  vacc_32bit/2(valid) -> real/3, Counter/2
  Counter/1 -> real/1
  Reinterpret/1 -> real/2

== system wb_poco_al_intfract_v00/dir_x/bd ==
  a+bi : Inport  Port=1  LatchInput=off
  c+di : Inport  Port=2  LatchInput=off
  new_acc : Inport  Port=3  LatchInput=off
  Counter : xbsIndex_r3/Counter  cnt_type=Free Running  n_bits=11  bin_pt=0  arith_type=Unsigned  start_count=0  cnt_to=Inf  cnt_by_val=1  operation=Up  explicit_period=off  period=1  load_pin=off  rst=on  en=on  dbl_ovrd=off  show_param=off  use_rpm=on  gen_core=off
      settings: xl_area=[0, 0, 0, 0, 0, 0, 0]
  Delay3 : xbsIndex_r3/Delay  latency=5  reg_retiming=off  explicit_period=off  period=1  en=off  accept_only_valid=off  init_zero=on  dbl_ovrd=off  show_param=off
      settings: xl_area=[0, 0, 0, 0, 0, 0, 0]
  Reinterpret : xbsIndex_r3/Reinterpret  force_arith_type=on  arith_type=Unsigned  force_bin_pt=on  bin_pt=0  force_valid=on
  Reinterpret1 : xbsIndex_r3/Reinterpret  force_arith_type=on  arith_type=Unsigned  force_bin_pt=on  bin_pt=0  force_valid=on
  c_to_ri : Subsystem  mask(Complex to Real-Imag){n_bits=4, bin_pt=3}
      mask prompts: n_bits "Bit Width"; bin_pt "Binary Point"
      mask help: Outputs real and imaginary components of a complex input.
      mask init:
      | annotation=sprintf('%d_%d r/i',n_bits,bin_pt);
      | set_param(gcb,'AttributesFormatString',annotation);
      settings: AttributesFormatString=4_3 r/i
      mask Help:
      | <pre>
      | Description::
      | 
      | Outputs real and imaginary components of a complex input.
      | Useful for simplifying interconnects.
      | See also: Real-Imag to Complex (ri_to_c)
      | 
      | Mask Parameters::
      | 
      | Bit Width (n_bits): Specifies the width of the real/imaginary components.
      | Assumed equal for both components.
      | 
      | Binary Point (bin_pt): Specifies the binary point location in the real/imaginary components.
      | Assumed equal for both components.
      | </pre>
  c_to_ri1 : Subsystem  mask(Complex to Real-Imag){n_bits=4, bin_pt=3}
      mask prompts: n_bits "Bit Width"; bin_pt "Binary Point"
      mask help: Outputs real and imaginary components of a complex input.
      mask init:
      | annotation=sprintf('%d_%d r/i',n_bits,bin_pt);
      | set_param(gcb,'AttributesFormatString',annotation);
      settings: AttributesFormatString=4_3 r/i
      mask Help:
      | <pre>
      | Description::
      | 
      | Outputs real and imaginary components of a complex input.
      | Useful for simplifying interconnects.
      | See also: Real-Imag to Complex (ri_to_c)
      | 
      | Mask Parameters::
      | 
      | Bit Width (n_bits): Specifies the width of the real/imaginary components.
      | Assumed equal for both components.
      | 
      | Binary Point (bin_pt): Specifies the binary point location in the real/imaginary components.
      | Assumed equal for both components.
      | </pre>
  cmult_4bit_sl* : Subsystem  mask(cmult_4bit_sl*){mult_latency=3, add_latency=2}
      mask prompts: mult_latency "Mult Latency"; add_latency "Add Latency"
      mask help: Perform a conjugating complex multiplication (a+bi)(c-di)=(ac+bd)+(bc-ad)i. Implements the logic in Slices.
      mask Help: eval('xlWeb([getenv(''MLIB_ROOT''), ''\doc\html\sp_cmult_4bit_sl_\sp_cmult_4bit_sl_.html''])')
  imag : xps_library/Shared BRAM  Tag=xps:bram  arith_type=Unsigned  addr_width=chan_bits+1  data_width=32  data_bin_pt=0  init_vals=0  sample_rate=1
  real : xps_library/Shared BRAM  Tag=xps:bram  arith_type=Unsigned  addr_width=chan_bits+1  data_width=32  data_bin_pt=0  init_vals=0  sample_rate=1
  vacc_0 : Subsystem  mask{n_chans=n_chans}
      mask prompts: n_chans "Number of channels"
      mask init:
      | chan_bits=ceil(log2(n_chans));
  vacc_1 : Subsystem  mask{n_chans=n_chans}
      mask prompts: n_chans "Number of channels"
      mask init:
      | chan_bits=ceil(log2(n_chans));
  wires:
  cmult_4bit_sl*/1(real) -> vacc_0/1(din)
  cmult_4bit_sl*/2(imag) -> vacc_1/1(din)
  c_to_ri/1(re) -> cmult_4bit_sl*/1(a)
  c_to_ri/2(im) -> cmult_4bit_sl*/2(b)
  c_to_ri1/1(re) -> cmult_4bit_sl*/3(c)
  c_to_ri1/2(im) -> cmult_4bit_sl*/4(d)
  a+bi/1 -> c_to_ri/1(c)
  c+di/1 -> c_to_ri1/1(c)
  Delay3/1 -> Counter/1, vacc_0/2(new_acc), vacc_1/2(new_acc)
  new_acc/1 -> Delay3/1
  vacc_0/1(dout) -> Reinterpret/1
  vacc_0/2(valid) -> Counter/2, real/3
  Reinterpret/1 -> real/2
  vacc_1/2(valid) -> imag/3
  Reinterpret1/1 -> imag/2
  vacc_1/1(dout) -> Reinterpret1/1
  Counter/1 -> imag/1, real/1
